simulink model "AMCLIB_FWSpeedLoop_BAM"  (Simulink 9.3)
settings: Solver=VariableStepAuto  StartTime=0.0  StopTime=10.0  RelTol=1e-3
(part 2 of 2)

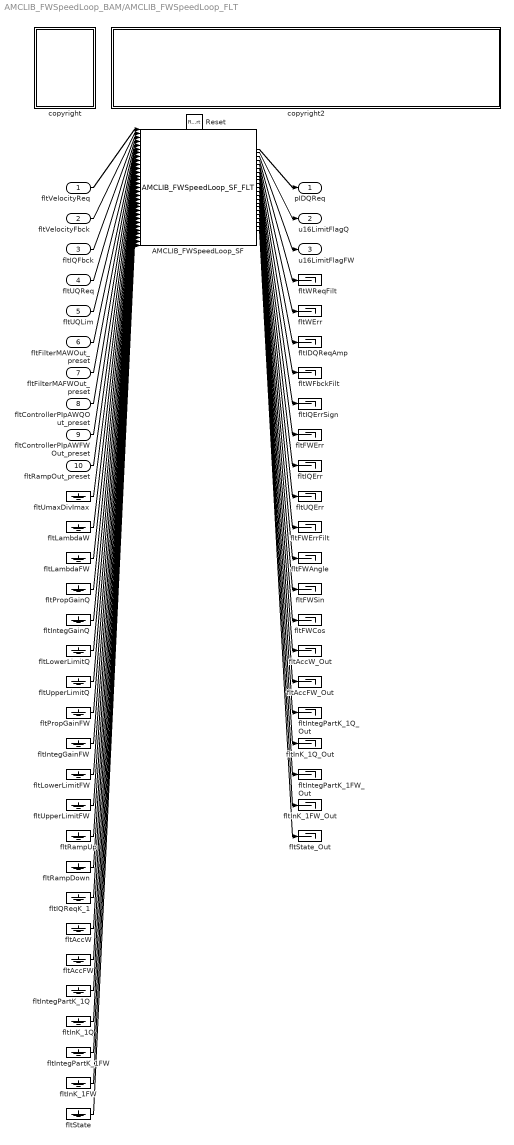
== system AMCLIB_FWSpeedLoop_BAM/AMCLIB_FWSpeedLoop_FLT ==
  fltVelocityReq : Inport  OutDataTypeStr=single
  fltVelocityFbck : Inport  Port=2  OutDataTypeStr=single
  fltIQFbck : Inport  Port=3  OutDataTypeStr=single
  fltUQReq : Inport  Port=4  OutDataTypeStr=single
  fltUQLim : Inport  Port=5  OutDataTypeStr=single
  fltFilterMAWOut_preset : Inport  Port=6  OutDataTypeStr=single
  fltFilterMAFWOut_preset : Inport  Port=7  OutDataTypeStr=single
  fltControllerPIpAWQOut_preset : Inport  Port=8  OutDataTypeStr=single
  fltControllerPIpAWFWOut_preset : Inport  Port=9  OutDataTypeStr=single
  fltRampOut_preset : Inport  Port=10  OutDataTypeStr=single
  Reset : ResetPort  DisableCoverage=on
  AMCLIB_FWSpeedLoop_SF : S-Function  FunctionName=AMCLIB_FWSpeedLoop_SF_FLT  Parameters=showStates,resetStatesEnable,showDebugOutputs,fltUmaxDivImax,fltLambdaW,fltLambdaFW,fltPropGainQ,fltIntegGainQ,fltLowerLimitQ,fltUpperLimitQ,fltPropGainFW,fltIntegGainFW,fltLowerLimitFW,fltUpperLimitFW,fltRampUp,fltRampDown  SFunctionDeploymentMode=off  EnableBusSupport=off
  copyright : Subsystem
      mask Display: text(10,90,'FILE:');text(10,75,'DESRIPTION:');text(10,60,'COPYRIGHT:');text(10,45,'VERSION:');text(10,30,'DATE:')
  copyright2 : Subsystem
      mask Display: text(10,90,'AMCLIB_FWSpeedLoop_BAM_FLT.mdl');text(10,75,'PMSM Speed Loop with Field Weakening.');text(10,60,'NXP 2020');text(10,45,'1.0');text(10,30,'28-Mar-2020');
  fltAccFW : Ground
  fltAccFW_Out : Terminator
  fltAccW : Ground
  fltAccW_Out : Terminator
  fltFWAngle : Terminator
  fltFWCos : Terminator
  fltFWErr : Terminator
  fltFWErrFilt : Terminator
  fltFWSin : Terminator
  fltIDQReqAmp : Terminator
  fltIQErr : Terminator
  fltIQErrSign : Terminator
  fltIQReqK_1 : Ground
  fltInK_1FW : Ground
  fltInK_1FW_Out : Terminator
  fltInK_1Q : Ground
  fltInK_1Q_Out : Terminator
  fltIntegGainFW : Ground
  fltIntegGainQ : Ground
  fltIntegPartK_1FW : Ground
  fltIntegPartK_1FW_Out : Terminator
  fltIntegPartK_1Q : Ground
  fltIntegPartK_1Q_Out : Terminator
  fltLambdaFW : Ground
  fltLambdaW : Ground
  fltLowerLimitFW : Ground
  fltLowerLimitQ : Ground
  fltPropGainFW : Ground
  fltPropGainQ : Ground
  fltRampDown : Ground
  fltRampUp : Ground
  fltState : Ground
  fltState_Out : Terminator
  fltUQErr : Terminator
  fltUmaxDivImax : Ground
  fltUpperLimitFW : Ground
  fltUpperLimitQ : Ground
  fltWErr : Terminator
  fltWFbckFilt : Terminator
  fltWReqFilt : Terminator
  pIDQReq : Outport
  u16LimitFlagQ : Outport  Port=2
  u16LimitFlagFW : Outport  Port=3
  wires:
  fltVelocityReq/1 -> AMCLIB_FWSpeedLoop_SF/1
  fltVelocityFbck/1 -> AMCLIB_FWSpeedLoop_SF/2
  fltIQFbck/1 -> AMCLIB_FWSpeedLoop_SF/3
  fltUQReq/1 -> AMCLIB_FWSpeedLoop_SF/4
  fltUQLim/1 -> AMCLIB_FWSpeedLoop_SF/5
  fltFilterMAWOut_preset/1 -> AMCLIB_FWSpeedLoop_SF/6
  fltFilterMAFWOut_preset/1 -> AMCLIB_FWSpeedLoop_SF/7
  fltControllerPIpAWQOut_preset/1 -> AMCLIB_FWSpeedLoop_SF/8
  fltControllerPIpAWFWOut_preset/1 -> AMCLIB_FWSpeedLoop_SF/9
  fltRampOut_preset/1 -> AMCLIB_FWSpeedLoop_SF/10
  fltUmaxDivImax/1 -> AMCLIB_FWSpeedLoop_SF/11
  fltLambdaW/1 -> AMCLIB_FWSpeedLoop_SF/12
  fltLambdaFW/1 -> AMCLIB_FWSpeedLoop_SF/13
  fltPropGainQ/1 -> AMCLIB_FWSpeedLoop_SF/14
  fltIntegGainQ/1 -> AMCLIB_FWSpeedLoop_SF/15
  fltLowerLimitQ/1 -> AMCLIB_FWSpeedLoop_SF/16
  fltUpperLimitQ/1 -> AMCLIB_FWSpeedLoop_SF/17
  fltPropGainFW/1 -> AMCLIB_FWSpeedLoop_SF/18
  fltIntegGainFW/1 -> AMCLIB_FWSpeedLoop_SF/19
  fltLowerLimitFW/1 -> AMCLIB_FWSpeedLoop_SF/20
  fltUpperLimitFW/1 -> AMCLIB_FWSpeedLoop_SF/21
  fltRampUp/1 -> AMCLIB_FWSpeedLoop_SF/22
  fltRampDown/1 -> AMCLIB_FWSpeedLoop_SF/23
  fltIQReqK_1/1 -> AMCLIB_FWSpeedLoop_SF/24
  fltAccW/1 -> AMCLIB_FWSpeedLoop_SF/25
  fltAccFW/1 -> AMCLIB_FWSpeedLoop_SF/26
  fltIntegPartK_1Q/1 -> AMCLIB_FWSpeedLoop_SF/27
  fltInK_1Q/1 -> AMCLIB_FWSpeedLoop_SF/28
  fltIntegPartK_1FW/1 -> AMCLIB_FWSpeedLoop_SF/29
  fltInK_1FW/1 -> AMCLIB_FWSpeedLoop_SF/30
  fltState/1 -> AMCLIB_FWSpeedLoop_SF/31
  AMCLIB_FWSpeedLoop_SF/1 -> pIDQReq/1
  AMCLIB_FWSpeedLoop_SF/2 -> u16LimitFlagQ/1
  AMCLIB_FWSpeedLoop_SF/3 -> u16LimitFlagFW/1
  AMCLIB_FWSpeedLoop_SF/4 -> fltWReqFilt/1
  AMCLIB_FWSpeedLoop_SF/5 -> fltWErr/1
  AMCLIB_FWSpeedLoop_SF/6 -> fltIDQReqAmp/1
  AMCLIB_FWSpeedLoop_SF/7 -> fltWFbckFilt/1
  AMCLIB_FWSpeedLoop_SF/8 -> fltIQErrSign/1
  AMCLIB_FWSpeedLoop_SF/9 -> fltFWErr/1
  AMCLIB_FWSpeedLoop_SF/10 -> fltIQErr/1
  AMCLIB_FWSpeedLoop_SF/11 -> fltUQErr/1
  AMCLIB_FWSpeedLoop_SF/12 -> fltFWErrFilt/1
  AMCLIB_FWSpeedLoop_SF/13 -> fltFWAngle/1
  AMCLIB_FWSpeedLoop_SF/14 -> fltFWSin/1
  AMCLIB_FWSpeedLoop_SF/15 -> fltFWCos/1
  AMCLIB_FWSpeedLoop_SF/16 -> fltAccW_Out/1
  AMCLIB_FWSpeedLoop_SF/17 -> fltAccFW_Out/1
  AMCLIB_FWSpeedLoop_SF/18 -> fltIntegPartK_1Q_Out/1
  AMCLIB_FWSpeedLoop_SF/19 -> fltInK_1Q_Out/1
  AMCLIB_FWSpeedLoop_SF/20 -> fltIntegPartK_1FW_Out/1
  AMCLIB_FWSpeedLoop_SF/21 -> fltInK_1FW_Out/1
  AMCLIB_FWSpeedLoop_SF/22 -> fltState_Out/1

== system AMCLIB_FWSpeedLoop_BAM/AMCLIB_FWSpeedLoop_FLT/copyright ==

== system AMCLIB_FWSpeedLoop_BAM/AMCLIB_FWSpeedLoop_FLT/copyright2 ==
